simulink model "DC_Generator"  (R2025a)
settings: Solver=ode23tb  StartTime=0.0  StopTime=10.0  MaxStep=1e-4  RelTol=1e-3
libraries: spsDCMachineLib x1, spsSeriesRLCBranchLib x1, spsDCVoltageSourceLib x1, spsVoltageMeasurementLib x1, sps_lib x1
settings Model: Creator=Jawad  LastModifiedBy=Jawad

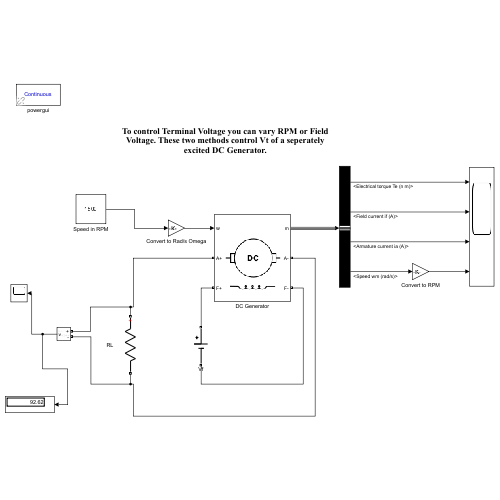
[thumbnail: Simulink's stored preview of the top-level diagram]
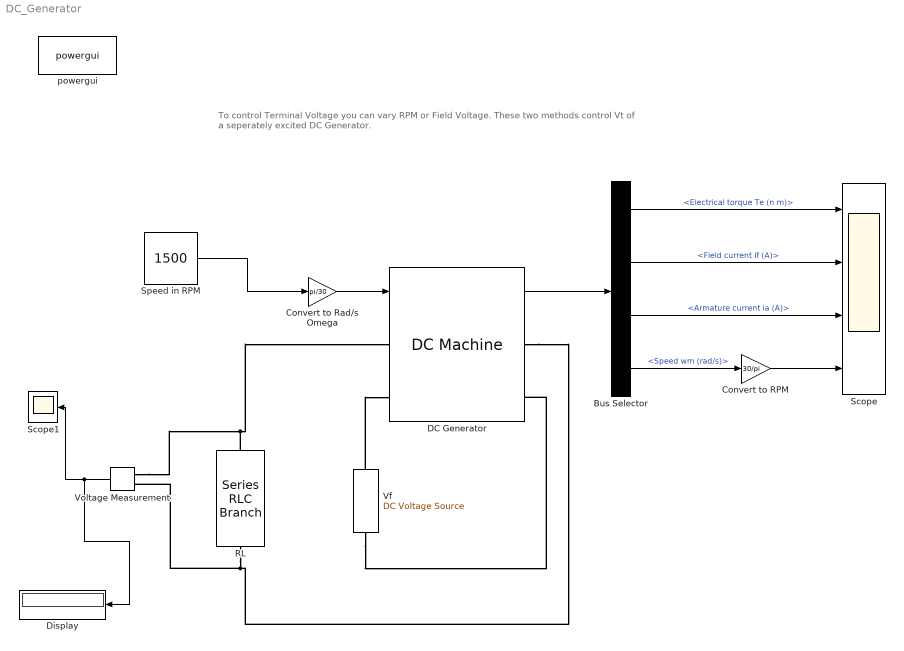
== system DC_Generator ==
  note: To control Terminal Voltage you can vary RPM or Field Voltage. These two methods control Vt of a seperately excited DC Generator.
  Bus Selector : BusSelector  OutputSignals=Electrical torque Te (n m),Field current if (A),Armature current ia (A),Speed wm (rad/s)
  Convert to RPM : Gain  Gain=30/pi
  Convert to Rad/s Omega : Gain  Gain=pi/30
  DC Generator : spsDCMachineLib/DC Machine  PresetModel=No  MechanicalLoad=Speed w  FieldType=Wound  ShowDetailedParameters=on  MeasurementBus=off  RLa="[ 0.6  0.012]"  RLf="[ 240  120]"  Laf=1.5  MachineConstant=Torque constant (N.m/A)  Ke=1.8  Kt=1.8  J=1  Bm=0  Tf=0  w0=1  Ifinit=0.416666666666667  TsPowergui=0  TsBlock=-1
  Display : Display
      settings: Decimation=2
  RL : spsSeriesRLCBranchLib/Series RLC Branch  LConnTagsString=__new0  RConnTagsString=__new0  BranchType=R  Resistance=10  Inductance=1e-3  SetiL0=off  InitialCurrent=0  Capacitance=1e-6  Setx0=off  InitialVoltage=0  Measurements=None
  Scope : Scope  NumInputPorts=4
      settings: ActiveDisplayYMinimum=-45.748230002523911  ActiveDisplayYMaximum=421.73512916702305
  Scope1 : Scope
      settings: ActiveDisplayYMinimum=55.532846634191486  ActiveDisplayYMaximum=239.47669668933304
  Speed in RPM : Constant  Value=1500
  Vf : spsDCVoltageSourceLib/DC Voltage Source  Amplitude=240  Measurements=None
  Voltage Measurement : spsVoltageMeasurementLib/Voltage Measurement  PhasorSimulation=off  OutputType=Complex  PSBequivalent=0
  powergui : sps_lib/powergui  Priority=1  SimulationMode=Continuous  SampleTime=50e-6  frequency=60  Iterations=50  frequencyindice=0  Pbase=100e6  ErrMax=1e-4  UnitsV=kV  UnitsW=MW  buscounter=0  FunctionMessages=off  echomessages=off  EnableUseOfTLC=off  CurrentSourceSwitches=off  DisableSnubberDevices=off  DisableRonSwitches=off  DisableVfSwitches=off  DisplayEquations=off  AutomaticDiscreteSolvers=off  SolverType=Tustin/Backward Euler (TBE)  Interpol=off  ExternalGateDelay=off  methode=off  Ts=100  x0status=blocks  SPID=on  SwTol=0  HookPort=off  NonlinearTolerance=1e-4  nMaxIteration=100  ContinueOnMaxIteration=off  RestoreLinks=warning  ResistiveCurrentMeasurement=off  Frange=[0:2:500]  Ylog=off  Xlog=on  ShowGrid=off  save=off  variable=ZData  structure=0  ZoomFFT=off  StartTime=0.0  cycles=1  DisplayStyle=1  fundamental=60  FreqAxis=off  MaxFrequency=1000  frequencyindicesteady=1  RmsSteady=1  display=off
  wires:
  Bus Selector/1 -> Scope/1  "<Electrical torque Te (n m)>"
  DC Generator/1 -> Bus Selector/1
  Bus Selector/3 -> Scope/3  "<Armature current ia (A)>"
  Bus Selector/4 -> Convert to RPM/1  "<Speed wm (rad/s)>"
  Convert to RPM/1 -> Scope/4
  Speed in RPM/1 -> Convert to Rad/s Omega/1
  Bus Selector/2 -> Scope/2  "<Field current if (A)>"
  Voltage Measurement/1 -> Display/1, Scope1/1
  Convert to Rad/s Omega/1 -> DC Generator/1
  connections:
  Voltage Measurement/LConn1 -- RL/LConn1 -- DC Generator/LConn1
  Vf/RConn1 -- DC Generator/LConn2
  Vf/LConn1 -- DC Generator/RConn2
  DC Generator/RConn1 -- RL/RConn1 -- Voltage Measurement/LConn2
